simulink model "mimiqua_leg2"  (R2022a)
settings: Solver=FixedStepAuto  StartTime=0.0  StopTime=5  RelTol=1e-3  EnableMultiTasking=on
undefined symbols (not defined in the file or in its folder): sigbuilder_block
libraries: raspberrypiCommlib x6, slpidlib x1
settings Model: Creator=wihsk  LastModifiedBy=drcl
settings SolverCC: PositivePriorityOrder=on
settings OptimizationCC: EnhancedBackFolding=on  PassReuseOutputArgsAs=Individual arguments  ZeroExternalMemoryAtStartup=off  ZeroInternalMemoryAtStartup=off  MaxStackSize=64  OptimizeBlockOrder=speed  DifferentSizesBufferReuse=on  OptimizationCustomize=off  EfficientTunableParamExpr=on
settings DebuggingCC: ParameterTunabilityLossMsg=error  UnconnectedInputMsg=warning  UnconnectedOutputMsg=warning  UnconnectedLineMsg=warning
settings HardwareCC: ProdBitPerPointer=32  ProdBitPerSizeT=32  ProdBitPerPtrDiffT=32  ProdLargestAtomicInteger=Long  ProdLargestAtomicFloat=Double  ProdWordSize=32  ProdLongLongMode=on  ProdHWDeviceType=ARM Compatible->ARM Cortex
settings SFSimCC: SimTargetLang=C++
settings RTWCC: SystemTargetFile=ert.tlc  HardwareBoard=Raspberry Pi  TLCOptions="-aInlineSetEventsForThisBaseRateFcn=TLC_TRUE -aSuppressMultiTaskScheduler=TLC_FALSE  -aRateBasedStepFcn=0"  TemplateMakefile=ert_default_tmf  Toolchain=GNU GCC Embedded Linux  BuildConfiguration=Faster Runs  TargetLang=C++  DLArmComputeVersion=19.05
settings CodeAppCC: ForceParamTrailComments=on  IgnoreCustomStorageClasses=off  OperatorAnnotations=on  SimulinkDataObjDesc=on  SFDataObjDesc=on  InsertBlockDesc=on
settings ERTTargetCC: TargetLangStandard=C++11 (ISO)  CodeInterfacePackaging=C++ class  SupportContinuousTime=on  SupportVariableSizeSignals=on  ExtModeTransport=2  ExtModeStaticAlloc=on  ExtModeMexFile=ext_xcp  ExtModeIntrfLevel=Level2 - Open  RootIOFormat=Structure reference

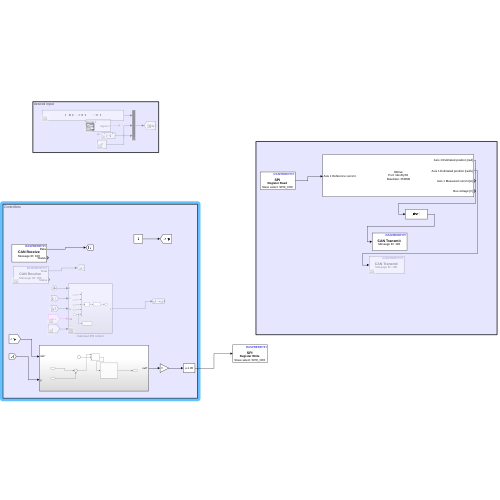
[thumbnail: Simulink's stored preview of the top-level diagram]
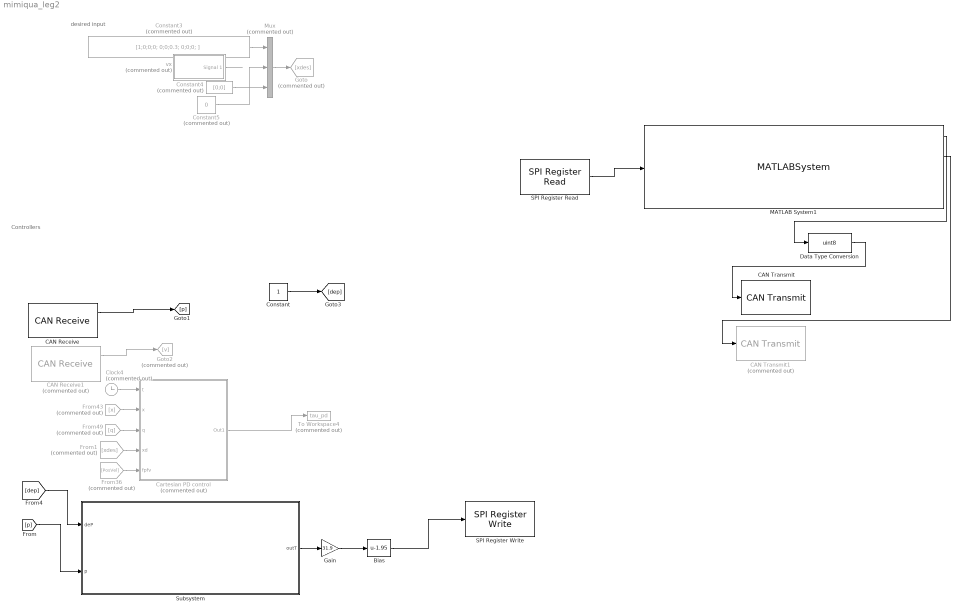
== system mimiqua_leg2 ==
  note: desired input
  note: Controllers
  Bias : Bias  Bias=-1.95  SaturateOnIntegerOverflow=off
  CAN Receive : raspberrypiCommlib/CAN Receive  DeviceID=can0  SetupCAN=off  TypeofCAN=Real  OutputDataType=Raw data  IdentifierType=Standard (11-bit identifier)  MessageId=100  MsgLength=8  SampleTime=-1  OutputError=off  OutputRemote=off  SimulateUsing=Code generation
      settings: SourceProductBaseCode=RASPPI
  CAN Receive1 : raspberrypiCommlib/CAN Receive  Commented=on  DeviceID=can0  SetupCAN=off  TypeofCAN=Real  OutputDataType=Raw data  IdentifierType=Standard (11-bit identifier)  MessageId=100  MsgLength=8  SampleTime=-1  OutputError=off  OutputRemote=off  SimulateUsing=Code generation
      settings: SourceProductBaseCode=RASPPI
  CAN Transmit : raspberrypiCommlib/CAN Transmit  DeviceID=can0  SetupCAN=off  TypeofCAN=Real  InputDataType=Raw data  BlockingMode_=off  BlockTimeout_=1  OutputStatus=off  IdentifierType=Standard (11-bit identifier)  MessageId=100  MsgLength=1  RemoteFrame=off  SimulateUsing=Code generation
      settings: SourceProductBaseCode=RASPPI
  CAN Transmit1 : raspberrypiCommlib/CAN Transmit  Commented=on  DeviceID=can0  SetupCAN=off  TypeofCAN=Real  InputDataType=Raw data  BlockingMode_=off  BlockTimeout_=1  OutputStatus=off  IdentifierType=Standard (11-bit identifier)  MessageId=100  MsgLength=8  RemoteFrame=off  SimulateUsing=Code generation
      settings: SourceProductBaseCode=RASPPI
  Cartesian PD control : Subsystem  Commented=on
  Clock4 : Clock  Commented=on
  Constant : Constant
  Constant3 : Constant  Commented=on  Value=[1;0;0;0; 0;0;0.3; 0;0;0; ]
  Constant4 : Constant  Commented=on  Value=[0;0]
  Constant5 : Constant  Commented=on  Value=0
  Data Type Conversion : DataTypeConversion  OutDataTypeStr=uint8  SaturateOnIntegerOverflow=off  RndMeth=Floor
  From1 : From  Commented=on  GotoTag=xdes
  From36 : From  Commented=on  GotoTag=PosVel
  From43 : From  Commented=on  GotoTag=x
  From49 : From  Commented=on  GotoTag=q
  Gain : Gain  Gain=31.9
  Goto : Goto  Commented=on  GotoTag=xdes
  Goto2 : Goto  Commented=on  GotoTag=v
  MATLAB System1 : MATLABSystem  System=ODrive  Port=/dev/ttyS0  Baudrate=250000  Autocalibration=Autocalibrate  EnableTiming=off  EnableAxis0=off  UseIndex0=on  ResetErrors0=on  ControlMode0=Current  VelocityLimit0=20*pi  CurrentLimit0=65  CountsPerRotate0=8192  EnablePosition0Output=on  EnableVelocity0Output=on  EnableCurrent0Output=on  EnableError0Output=off  EnableAxis1=on  UseIndex1=on  ResetErrors1=on  ControlMode1=Current  VelocityLimit1=20*pi  CurrentLimit1=20  CountsPerRotate1=8192  EnablePosition1Output=on  EnableVelocity1Output=on  EnableCurrent1Output=on  EnableError1Output=off  MaxInputParameters=20  Inputs={}  MaxOutputParameters=20  EnableVbusOutput=on  Outputs="{  }"
      mask Type: ODrive
      mask Display:
      | disp(['ODrive' char(10) 'Port: /dev/ttyS0' char(10) ' Baudrate: 250000']);
      | port_label('input',1,'Axis 1 Reference current');
      | port_label('output',1,'Axis 1 Estimated position [rad]');
      | port_label('output',2,'Axis 1 Estimated position [rad/s]');
      | port_label('output',3,'Axis 1 Measured current [A]');
      | port_label('output',4,'Bus voltage [V]');
  Mux : Mux  Commented=on  Inputs=3
  SPI Register Read : raspberrypiCommlib/SPI Register Read  BoardProperty=Pi 3 Model B+  SSPin=SPI0_CE0  SPIModule=uint32(0)  Mode=Master  BusSpeed=1000000  Pin=uint32(0)  FirstBitToTransfer=Most significant bit (MSB)  ClockMode=0  BlockFunction=Read  RegisterAddress=0  OutputDataType=double  OutputDataLength=1  SampleTime=0.1
      settings: SourceProductBaseCode=RASPPI
  SPI Register Write : raspberrypiCommlib/SPI Register Write  BoardProperty=Pi 3 Model B+  SSPin=SPI0_CE0  SPIModule=uint32(0)  Mode=Master  BusSpeed=1000000  Pin=uint32(0)  FirstBitToTransfer=Most significant bit (MSB)  ClockMode=0  BlockFunction=Write  RegisterAddress=0  OutputDataType=int8  OutputDataLength=1
      settings: SourceProductBaseCode=RASPPI
  Subsystem : Subsystem
  To Workspace4 : ToWorkspace  Commented=on  VariableName=tau_pd  SampleTime=-1
  vx : Subsystem  Tag=STV Subsys  Commented=on  LoadFcn=sigbuilder_block('load');  StartFcn=sigbuilder_block('start');  StopFcn=sigbuilder_block('stop');  ClipboardFcn=sigbuilder_block('clipboard');  mask(Sigbuilder block){tuvar=[0:10]}
      mask help: Simulink:masks:SigbuilderBlock_MD
      mask init:
      | if ~strcmp(get_param(bdroot(gcbh),'SimulationStatus'),'stopped') tuvar = sigbuilder_block('maskInit'); end
      settings: CopyFcn=sigbuilder_block('copy');  DeleteFcn=sigbuilder_block('delete');  ModelCloseFcn=sigbuilder_block('modelClose');  PreSaveFcn=sigbuilder_block('preSave');  PauseFcn=sigbuilder_block('pause');  ContinueFcn=sigbuilder_block('continue');  NameChangeFcn=sigbuilder_block('namechange');  OpenFcn=sigbuilder_block('open',[437.6 199.2 550.4 400 ]);  CloseFcn=sigbuilder_block('close');
      mask Display: plot(0, 0, 100, 100,[2, 2, 32, 32, 2], [68, 8, 8, 68, 68],[32, 2], [38, 38], [32, 19, 2],[53, 60, 44], [32, 17, 17, 2],[16, 16, 31, 31]);txt = getActiveGroup(gcbh);text(2, 100, txt,'verticalAlignment', 'top');
  wires:
  Constant4/1 -> Mux/3
  Constant5/1 -> Mux/2
  Mux/1 -> Goto/1
  vx/1(Signal 1) -> ?
  Constant3/1 -> Mux/1
  Cartesian PD control/1(Out1) -> To Workspace4/1
  Clock4/1 -> Cartesian PD control/1(t)
  From49/1 -> Cartesian PD control/3(q)
  From36/1 -> Cartesian PD control/5(fpfv)
  From43/1 -> Cartesian PD control/2(x)
  From1/1 -> Cartesian PD control/4(xd)
  MATLAB System1/2 -> CAN Transmit1/1
  SPI Register Read/1 -> MATLAB System1/1
  CAN Receive/1 -> [p]
  CAN Receive1/1 -> Goto2/1
  [p] -> Subsystem/2(p)
  [dep] -> Subsystem/1(deP)
  Subsystem/1(outT) -> Gain/1
  Gain/1 -> Bias/1
  Bias/1 -> SPI Register Write/1
  Constant/1 -> [dep]
  MATLAB System1/1 -> Data Type Conversion/1
  Data Type Conversion/1 -> CAN Transmit/1

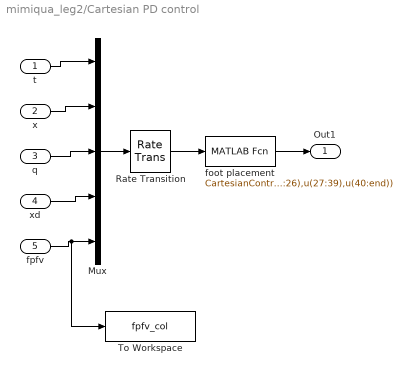
== system mimiqua_leg2/Cartesian PD control ==
  t : Inport
  x : Inport  Port=2
  q : Inport  Port=3
  xd : Inport  Port=4
  fpfv : Inport  Port=5
  Mux : Mux  Inputs=5
  Rate Transition : RateTransition  OutPortSampleTime=0.001
  To Workspace : ToWorkspace  VariableName=fpfv_col  SampleTime=-1
  foot placement : MATLABFcn  MATLABFcn=CartesianControl(u(1),u(2:14),u(15:26),u(27:39),u(40:end))  OutputDimensions=[12 1]  Output1D=off
  Out1 : Outport
  wires:
  t/1 -> Mux/1
  x/1 -> Mux/2
  xd/1 -> Mux/4
  q/1 -> Mux/3
  fpfv/1 -> To Workspace/1, Mux/5
  Mux/1 -> Rate Transition/1
  foot placement/1 -> Out1/1
  Rate Transition/1 -> foot placement/1

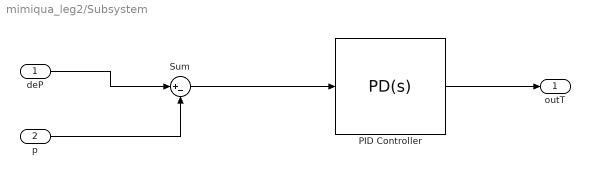
== system mimiqua_leg2/Subsystem ==
  deP : Inport
  p : Inport  Port=2
  PID Controller : slpidlib/PID Controller  Controller=PD  Form=Parallel  TimeDomain=Continuous-time  UseExternalTs=off  SampleTime=-1  IntegratorMethod=Forward Euler  FilterMethod=Forward Euler  ControllerParametersSource=internal  P=1  I=0  UseKiTs=off  D=1  N=100  UseFilter=on  TunerSelectOption=Transfer Function Based (PID Tuner App)  InitialConditionSource=internal  InitialConditionForIntegrator=0  InitialConditionForFilter=0  DifferentiatorICPrevScaledInput=0  ExternalReset=none  TrackingMode=off  Kt=1  LimitOutput=off  SatLimitsSource=internal  UpperSaturationLimit=inf  LowerSaturationLimit=-inf  LinearizeAsGain=on  AntiWindupMode=none  Kb=1  POutMin=[]  POutMax=[]  IOutMin=[]  IOutMax=[]  DOutMin=[]  DOutMax=[]  NOutMin=[]  NOutMax=[]  SumOutMin=[]  SumOutMax=[]  SaturationOutMin=[]  SaturationOutMax=[]  PParamMin=[]  PParamMax=[]  IParamMin=[]  IParamMax=[]  DParamMin=[]  DParamMax=[]  NParamMin=[]  NParamMax=[]  KbParamMin=[]  KbParamMax=[]  KtParamMin=[]  KtParamMax=[]  KbOutMin=[]  KbOutMax=[]  KtOutMin=[]  KtOutMax=[]  IntegratorOutMin=[]  IntegratorOutMax=[]  FilterOutMin=[]  FilterOutMax=[]  SumI1OutMin=[]  SumI1OutMax=[]  SumI2OutMin=[]  SumI2OutMax=[]  SumI3OutMin=[]  SumI3OutMax=[]  SumI4OutMin=[]  SumI4OutMax=[]  SumDOutMin=[]  SumDOutMax=[]  DifferentiatorOutMin=[]  DifferentiatorOutMax=[]  FilterDiffOutCoefMin=[]  FilterDiffOutCoefMax=[]  ReciprocalOutMin=[]  ReciprocalOutMax=[]  SumDenOutMin=[]  SumDenOutMax=[]  SumNumOutMin=[]  SumNumOutMax=[]  DivideOutMin=[]  DivideOutMax=[]  UdiffTsProdOutMin=[]  UdiffTsProdOutMax=[]  NTsProdOutMin=[]  NTsProdOutMax=[]  UintegralTsProdOutMin=[]  UintegralTsProdOutMax=[]  UngainTsProdOutMin=[]  UngainTsProdOutMax=[]  IntegratorContinuousStateAttributes=''  IntegratorStateMustResolveToSignalObject=off  IntegratorRTWStateStorageClass=Auto  FilterContinuousStateAttributes=''  FilterStateMustResolveToSignalObject=off  FilterRTWStateStorageClass=Auto  ParallelPVariant=InternalParameters  IdealPVariant=Disabled  IVariant=Disabled  DVariant=InternalParameters  IntegratorVariant=Disabled  SatVariant=Disabled  AWVariant=Disabled  PCopyVariant=Disabled  TRVariant=Disabled  FdbkBlocksVariant=Forward  IdealPFdbkVariant=Disabled  SatFdbkVariant=Disabled  DerivativeFilterVariant=ContFilter  NVariant=InternalParameters  NCopyVariant=Disabled  FilterICVariant=InternalICsFilter  IntegratorICVariant=Disabled  ExternalResetVariant=Disabled  TRSumVariant=Passthrough  SumFdbkVariant=Disabled  SumVariant=Sum_PD  TsampFilterVariant=InternalTs  TsampNgainVariant=Passthrough  TsampIntegralVariant=Disabled_SignalSpec  ExternalSaturationOutDataTypeStr=Inherit: Same as second input  aMode=0
  Sum : Sum  Inputs=|+-
  outT : Outport
  wires:
  deP/1 -> Sum/1
  p/1 -> Sum/2
  PID Controller/1 -> outT/1
  Sum/1 -> PID Controller/1

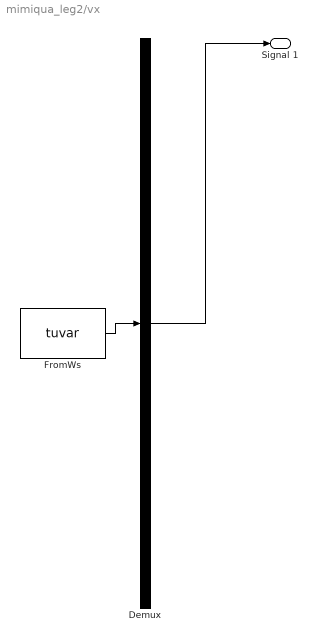
== system mimiqua_leg2/vx ==
  Demux : Demux  Tag=STV Demux  Outputs=1
      settings: DisplayOption=none
  FromWs : FromWorkspace  Tag=STV FromWs  VariableName=tuvar
      SigBuilderData=|
      | common.afterFinalStr = 'Extrapolate'
      | common.sampleTime = 0
      | dataSet.timeRange = [0 10]
      | dataSet.name = 'Group 1'
      | sbobj.Groups.Name = 'Group 1'
      | sbobj.Groups.Signals.Name = 'Signal 1'
      | sbobj.Groups.Signals.XData = [0 2 3 5 10]
      | sbobj.Groups.Signals.YData = [0 0.5 0.5 0.5 0]
  Signal 1 : Outport  Tag=STV Outport
  wires:
  Demux/1 -> Signal 1/1
  FromWs/1 -> Demux/1
